simulink model "DS_distrIntp_4_0_realaxes"  (R2019b)
settings: Solver=FixedStepDiscrete  StartTime=0.0  StopTime=inf  FixedStep=Ts  RelTol=1e-3
StartFcn:
  | close all;
model workspace (MAT data in the model file):
  MvmtPerfEval_collectVal = Simulink.Parameter
  MvmtPerfEval_collectVal.Value = 0.65
  MvmtPerfEval_collectVal.Description = '- Anteil eines Interpolationssegments (0,1)
    | - Nach Abarbeitung des spezifizierten Anteils wird gemeinsame Performance aller Agenten
    | vom Dispatcher geladen
    | 
    | - (!!!) Wert MUSS größer sein als MvmtPerfEval_sendOwnVal'
  MvmtPerfEval_collectVal.DataType = 'auto'
  MvmtPerfEval_collectVal.Min = 0
  MvmtPerfEval_collectVal.Max = 1
  MvmtPerfEval_collectVal.Dimensions = [1 1]
  MvmtPerfEval_sendOwnVal = Simulink.Parameter
  MvmtPerfEval_sendOwnVal.Value = 0.6
  MvmtPerfEval_sendOwnVal.Description = '- Anteil eines Interpolationssegments (0,1)
    | - Nach Abarbeitung des spezifizierten Anteils wird Perfomance Kennzahl an Dispatcher übermittelt
    | 
    | - (!!!) Wert MUSS kleiner sein als MvmtPerfEval_collectVal'
  MvmtPerfEval_sendOwnVal.DataType = 'auto'
  MvmtPerfEval_sendOwnVal.Min = 0
  MvmtPerfEval_sendOwnVal.Max = 1
  MvmtPerfEval_sendOwnVal.Dimensions = [1 1]
  PAR_center_c2 = Simulink.Parameter
  PAR_center_c2.Value = [0.0775 0.062 0.05]
  PAR_center_c2.DataType = 'double'
  PAR_center_c2.Dimensions = [1 3]
  PAR_numStepsAheadSmoothing = Simulink.Parameter
  PAR_numStepsAheadSmoothing.Value = 1
  PAR_numStepsAheadSmoothing.Description = 'Anzahl der Zeitschritte (Ts) vor Segmentende, welches Zeitpunkt festlegt,
    | an dem der kommende Verfahrbefehl gesendet wird'
  PAR_numStepsAheadSmoothing.DataType = 'auto'
  PAR_numStepsAheadSmoothing.Dimensions = [1 1]
  PAR_startPosReachedTol = Simulink.Parameter
  PAR_startPosReachedTol.Value = 0.002
  PAR_startPosReachedTol.DataType = 'auto'
  PAR_startPosReachedTol.Dimensions = [1 1]
  PAR_workspace_c2 = Simulink.Parameter
  PAR_workspace_c2.Value = [0 0 0.05 0.052 0.072]
  PAR_workspace_c2.DataType = 'double'
  PAR_workspace_c2.Dimensions = [1 5]
  PerfEval_numTicks_enable = Simulink.Parameter
  PerfEval_numTicks_enable.Value = 10
  PerfEval_numTicks_enable.Description = 'Anzahl der Ticks (Integrationsschritte), bevor die Performance ausgewertet wird
    | (unabhängig vom Senden des Werts an den Dispatcher)'
  PerfEval_numTicks_enable.DataType = 'auto'
  PerfEval_numTicks_enable.Dimensions = [1 1]
  Segmentregler_I_Gain = Simulink.Parameter
  Segmentregler_I_Gain.Value = 1
  Segmentregler_I_Gain.DataType = 'auto'
  Segmentregler_I_Gain.Dimensions = [1 1]
  Segmentregler_P_Gain = Simulink.Parameter
  Segmentregler_P_Gain.Value = 0
  Segmentregler_P_Gain.DataType = 'auto'
  Segmentregler_P_Gain.Dimensions = [1 1]
  Segmentregler_minVel_enable = Simulink.Parameter
  Segmentregler_minVel_enable.Value = 0.1
  Segmentregler_minVel_enable.DataType = 'auto'
  Segmentregler_minVel_enable.Dimensions = [1 1]
  Segmentregler_numTicks_enable = Simulink.Parameter
  Segmentregler_numTicks_enable.Value = 30
  Segmentregler_numTicks_enable.Description = 'Anzahl der Ticks (Integrationsschritte), bevor der Segmentregler aktiv wird'
  Segmentregler_numTicks_enable.DataType = 'auto'
  Segmentregler_numTicks_enable.Dimensions = [1 1]
  Ts = Simulink.Parameter
  Ts.Value = 0.005
  Ts.Description = 'Sampling Time'
  Ts.DataType = 'auto'
  Ts.Dimensions = [1 1]
  horizon = Simulink.Parameter
  horizon.Value = 0
  horizon.DataType = 'auto'
  horizon.Dimensions = [1 1]
  maxPos_x = Simulink.Parameter
  maxPos_x.Value = 300
  maxPos_x.Description = 'Grenze des Arbeitsbereichs (maximaler Wert der Koordinate)'
  maxPos_x.DataType = 'auto'
  maxPos_x.Dimensions = [1 1]
  maxPos_y = Simulink.Parameter
  maxPos_y.Value = 150
  maxPos_y.Description = 'Grenze des Arbeitsbereichs (maximaler Wert der Koordinate)'
  maxPos_y.DataType = 'auto'
  maxPos_y.Dimensions = [1 1]
  maxPos_z = Simulink.Parameter
  maxPos_z.Value = 50
  maxPos_z.Description = 'Grenze des Arbeitsbereichs (maximaler Wert der Koordinate)'
  maxPos_z.DataType = 'auto'
  maxPos_z.Dimensions = [1 1]
  maxVectorLengths = Simulink.Parameter
  maxVectorLengths.Value = 100000
  maxVectorLengths.DataType = 'auto'
  maxVectorLengths.Dimensions = [1 1]
  minAllowedVelSaturation = Simulink.Parameter
  minAllowedVelSaturation.Value = 0.25
  minAllowedVelSaturation.Description = 'Minimaler Saturation-Wert für den Geschwindigkeits-PID-Regler
    | (auch bei Sollgeschwindigkeit soll Fehlerkorrektur möglich sein)'
  minAllowedVelSaturation.DataType = 'auto'
  minAllowedVelSaturation.Dimensions = [1 1]
  numAxes = Simulink.Parameter
  numAxes.Value = 4
  numAxes.DataType = 'auto'
  numAxes.Dimensions = [1 1]
  window_length = Simulink.Parameter
  window_length.Value = 50
  window_length.DataType = 'auto'
  window_length.Dimensions = [1 1]
undefined symbols (not defined in the file or in its folder): DiscIntNeverNeededParam, setP_mat, VelOverride
libraries: vrlib x1, sldrtlib x1
(part 1 of 4)
settings Model: OrderedModelArguments=off  Creator=Daniel  LastModifiedBy=MAHFOUZ
settings DataIOCC: SignalLogging=off  ReturnWorkspaceOutputs=off
settings DebuggingCC: ArithmeticOperatorsInVariantConditions=warning
settings SFSimCC: CustomCodeUndefinedFunction=UseInterfaceOnly

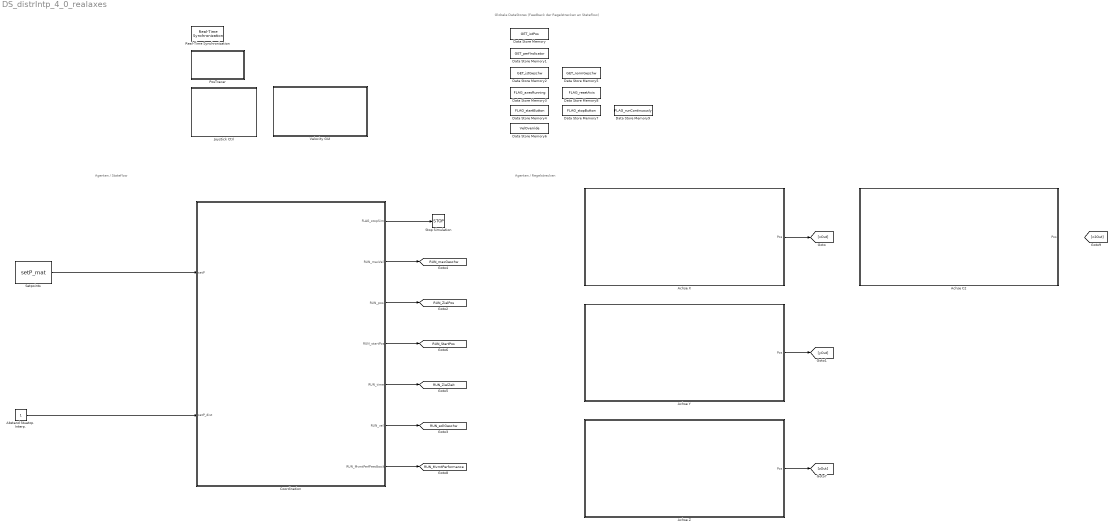
== system DS_distrIntp_4_0_realaxes ==
  note: Globale DataStores (Feedback der Regelstrecken an Stateflow)
  note: Agenten / Regelstrecken
  note: Agenten / Stateflow
  Abstand Stuetzp. Interp. : Constant
  Achse C2 : Subsystem
  Achse X : Subsystem
  Achse Y : Subsystem
  Achse Z : Subsystem
  Coordination : Stateflow chart  TreatAsAtomicUnit=on
  Data Store Memory : DataStoreMemory  DataStoreName=GET_istPos  ReadBeforeWriteMsg=warning  WriteAfterWriteMsg=warning  WriteAfterReadMsg=warning  InitialValue=zeros(1,numAxes)  ShowAdditionalParam=off  OutDataTypeStr=double
  Data Store Memory1 : DataStoreMemory  DataStoreName=GET_perfIndicator  ReadBeforeWriteMsg=warning  WriteAfterWriteMsg=warning  WriteAfterReadMsg=warning  InitialValue=zeros(1,numAxes)  ShowAdditionalParam=off  OutDataTypeStr=double
  Data Store Memory2 : DataStoreMemory  DataStoreName=GET_istGeschw  ReadBeforeWriteMsg=warning  WriteAfterWriteMsg=warning  WriteAfterReadMsg=warning  InitialValue=zeros(1,numAxes)  ShowAdditionalParam=off  OutDataTypeStr=double
  Data Store Memory3 : DataStoreMemory  DataStoreName=FLAG_axesRunning  ReadBeforeWriteMsg=warning  WriteAfterWriteMsg=warning  WriteAfterReadMsg=warning  InitialValue=false  ShowAdditionalParam=off  OutDataTypeStr=boolean
  Data Store Memory4 : DataStoreMemory  DataStoreName=FLAG_startButton  ReadBeforeWriteMsg=warning  WriteAfterWriteMsg=warning  WriteAfterReadMsg=warning  InitialValue=false  ShowAdditionalParam=off  OutDataTypeStr=boolean
  Data Store Memory5 : DataStoreMemory  DataStoreName=GET_normGeschw  ReadBeforeWriteMsg=warning  WriteAfterWriteMsg=warning  WriteAfterReadMsg=warning  InitialValue=zeros(1,numAxes)  ShowAdditionalParam=off  OutDataTypeStr=double
  Data Store Memory6 : DataStoreMemory  DataStoreName=VelOverride  ReadBeforeWriteMsg=warning  WriteAfterWriteMsg=warning  WriteAfterReadMsg=warning  InitialValue=ones(1,numAxes)  ShowAdditionalParam=off  OutDataTypeStr=double
  Data Store Memory7 : DataStoreMemory  DataStoreName=FLAG_stopButton  ReadBeforeWriteMsg=warning  WriteAfterWriteMsg=warning  WriteAfterReadMsg=warning  InitialValue=false  ShowAdditionalParam=off  OutDataTypeStr=boolean
  Data Store Memory8 : DataStoreMemory  DataStoreName=FLAG_resetAxis  ReadBeforeWriteMsg=warning  WriteAfterWriteMsg=warning  WriteAfterReadMsg=warning  InitialValue=zeros(1,numAxes)  ShowAdditionalParam=off  OutDataTypeStr=boolean
  Data Store Memory9 : DataStoreMemory  DataStoreName=FLAG_runContinuously  ReadBeforeWriteMsg=warning  WriteAfterWriteMsg=warning  WriteAfterReadMsg=warning  ShowAdditionalParam=off  OutDataTypeStr=double
  Joystick Ctrl : Subsystem
  PosTracer : Stateflow chart  BlockKeywords=__PRM__SERIALIZED__DATA__:Stateflow Chart,Stateflow Diagram  TreatAsAtomicUnit=on
  Real-Time Synchronization : sldrtlib/Real-Time Synchronization  SampleTime=0.005  MaxMissedTicks=2000  ShowMissedTicks=off  YieldWhenWaiting=off
  Setpoints : Constant  Value=setP_mat
  Stop Simulation : Stop
  Velocity GUI : Subsystem
  tag scope: RUN_MvmtPerformance=global, RUN_StartPos=global, RUN_ZielPos=global, RUN_ZielZeit=global, RUN_maxGeschw=global, RUN_sollGeschw=global
  wires:
  Abstand Stuetzp. Interp./1 -> Coordination/2(setP_dist)
  Setpoints/1 -> Coordination/1(setP)
  Coordination/2(RUN_maxVel) -> [RUN_maxGeschw]
  Coordination/3(RUN_pos) -> [RUN_ZielPos]
  Coordination/4(RUN_startPos) -> [RUN_StartPos]
  Coordination/5(RUN_time) -> [RUN_ZielZeit]
  Coordination/6(RUN_vel) -> [RUN_sollGeschw]
  Achse Z/1(Pos) -> [zOut]
  Coordination/7(RUN_MvmtPerfFeedback) -> [RUN_MvmtPerformance]
  Achse X/1(Pos) -> [xOut]
  Achse Y/1(Pos) -> [yOut]
  ? -> [c2Out]
  Coordination/1(FLAG_stopSim) -> Stop Simulation/1

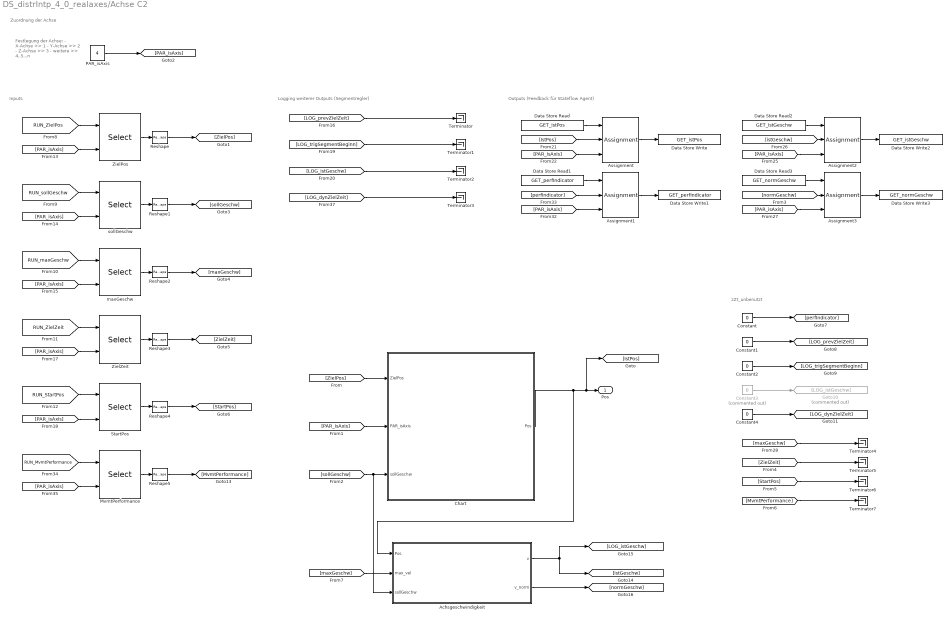
== system DS_distrIntp_4_0_realaxes/Achse C2 ==
  note: Outputs (Feedback für Stateflow Agent)
  note: Logging weiterer Outputs (Segmentregler)
  note: Zuordnung der Achse
  note: Festlegung der Achse:
      | - X-Achse >> 1
      | - Y-Achse >> 2
      | - Z-Achse >> 3
      | - weitere >> 4..5...n
  note: Inputs
  note: zZt_unbenutzt
  Achsgeschwindigkeit : Stateflow chart  BlockKeywords=__PRM__SERIALIZED__DATA__:Stateflow Chart,Stateflow Diagram  TreatAsAtomicUnit=on
  Assignment{,1..3} (4 alike) : Assignment  DiagnosticForDimensions=Warning  IndexOptions=Index vector (port)  Indices=1  OutputSizes=1
  Chart : Stateflow chart  BlockKeywords=__PRM__SERIALIZED__DATA__:Stateflow Chart,Stateflow Diagram  TreatAsAtomicUnit=on
  Constant{,1..2,4} (4 alike) : Constant  Value=0
  Constant3 : Constant  Commented=on  Value=0
  Data Store Read : DataStoreRead  DataStoreName=GET_istPos
  Data Store Read1 : DataStoreRead  DataStoreName=GET_perfIndicator
  Data Store Read2 : DataStoreRead  DataStoreName=GET_istGeschw
  Data Store Read3 : DataStoreRead  DataStoreName=GET_normGeschw
  Data Store Write : DataStoreWrite  DataStoreName=GET_istPos
  Data Store Write1 : DataStoreWrite  DataStoreName=GET_perfIndicator
  Data Store Write2 : DataStoreWrite  DataStoreName=GET_istGeschw
  Data Store Write3 : DataStoreWrite  DataStoreName=GET_normGeschw
  Goto10 : Goto  Commented=on  GotoTag=LOG_istGeschw
  MvmtPerformance : Selector  IndexOptions=Index vector (port)  Indices=[1 3]  OutputSizes=1
  PAR_isAxis : Constant  Value=4
  Reshape{,1..5} (6 alike) : Reshape
  StartPos : Selector  IndexOptions=Index vector (port)  Indices=[1 3]  OutputSizes=1
  Terminator{,1..7} (8 alike) : Terminator
  ZielPos : Selector  IndexOptions=Index vector (port)  Indices=[1 3]  OutputSizes=1
  ZielZeit : Selector  IndexOptions=Index vector (port)  Indices=[1 3]  OutputSizes=1
  maxGeschw : Selector  IndexOptions=Index vector (port)  Indices=[1 3]  OutputSizes=1
  sollGeschw : Selector  IndexOptions=Index vector (port)  Indices=[1 3]  OutputSizes=1
  Pos : Outport  VectorParamsAs1DForOutWhenUnconnected=off
  wires:
  PAR_isAxis/1 -> [PAR_isAxis]
  [PAR_isAxis] -> ZielPos/2
  [RUN_ZielPos] -> ZielPos/1
  ZielPos/1 -> Reshape/1
  sollGeschw/1 -> Reshape1/1
  [RUN_sollGeschw] -> sollGeschw/1
  [PAR_isAxis] -> sollGeschw/2
  [PAR_isAxis] -> maxGeschw/2
  [RUN_maxGeschw] -> maxGeschw/1
  maxGeschw/1 -> Reshape2/1
  ZielZeit/1 -> Reshape3/1
  [RUN_ZielZeit] -> ZielZeit/1
  [PAR_isAxis] -> ZielZeit/2
  [PAR_isAxis] -> StartPos/2
  [RUN_StartPos] -> StartPos/1
  StartPos/1 -> Reshape4/1
  [LOG_prevZielZeit] -> Terminator/1
  [LOG_trigSegmentBeginn] -> Terminator1/1
  [LOG_istGeschw] -> Terminator2/1
  Reshape/1 -> [ZielPos]
  Reshape1/1 -> [sollGeschw]
  Reshape2/1 -> [maxGeschw]
  Reshape4/1 -> [StartPos]
  Reshape3/1 -> [ZielZeit]
  Data Store Read/1 -> Assignment/1
  [IstPos] -> Assignment/2
  [PAR_isAxis] -> Assignment/3
  Assignment/1 -> Data Store Write/1
  Assignment1/1 -> Data Store Write1/1
  [PAR_isAxis] -> Assignment1/3
  [perfIndicator] -> Assignment1/2
  Data Store Read1/1 -> Assignment1/1
  Reshape5/1 -> [MvmtPerformance]
  MvmtPerformance/1 -> Reshape5/1
  [RUN_MvmtPerformance] -> MvmtPerformance/1
  [PAR_isAxis] -> MvmtPerformance/2
  [LOG_dynZielZeit] -> Terminator3/1
  Constant4/1 -> [LOG_dynZielZeit]
  Constant1/1 -> [LOG_prevZielZeit]
  [StartPos] -> Terminator6/1
  Constant2/1 -> [LOG_trigSegmentBeginn]
  [ZielZeit] -> Terminator5/1
  Constant/1 -> [perfIndicator]
  Constant3/1 -> Goto10/1
  [maxGeschw] -> Terminator4/1
  [MvmtPerformance] -> Terminator7/1
  [ZielPos] -> Chart/1(ZielPos)
  [PAR_isAxis] -> Chart/2(PAR_isAxis)
  [sollGeschw] -> Achsgeschwindigkeit/3(sollGeschw), Chart/3(sollGeschw)
  Chart/1(Pos) -> Achsgeschwindigkeit/1(Pos), Pos/1, [IstPos]
  Achsgeschwindigkeit/1(v) -> [istGeschw], [LOG_istGeschw]
  [normGeschw] -> Assignment3/2
  [istGeschw] -> Assignment2/2
  [PAR_isAxis] -> Assignment2/3
  [PAR_isAxis] -> Assignment3/3
  Assignment3/1 -> Data Store Write3/1
  Assignment2/1 -> Data Store Write2/1
  Data Store Read2/1 -> Assignment2/1
  Data Store Read3/1 -> Assignment3/1
  Achsgeschwindigkeit/2(v_norm) -> [normGeschw]
  [maxGeschw] -> Achsgeschwindigkeit/2(max_vel)

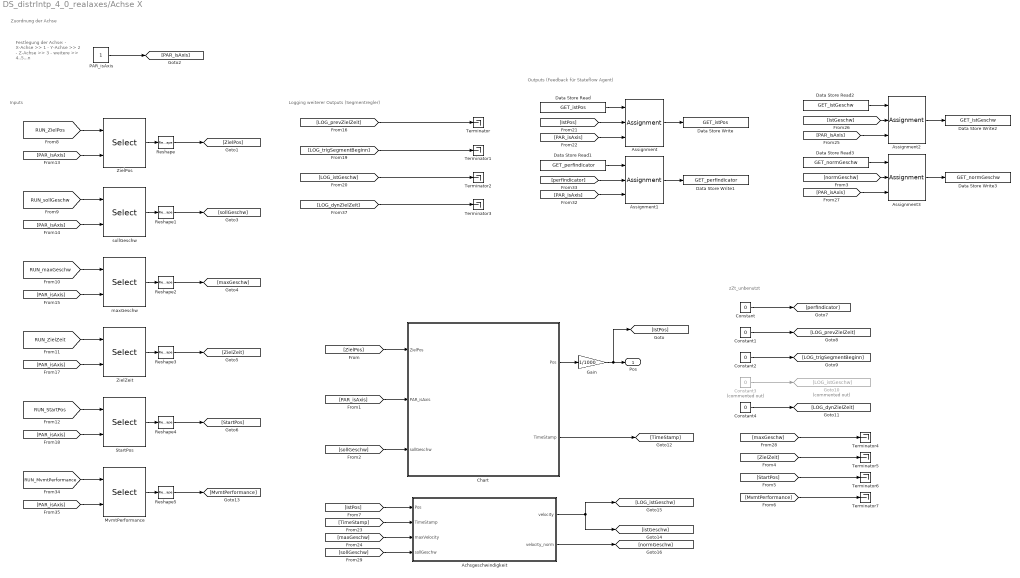
== system DS_distrIntp_4_0_realaxes/Achse X ==
  note: zZt_unbenutzt
  note: Outputs (Feedback für Stateflow Agent)
  note: Logging weiterer Outputs (Segmentregler)
  note: Zuordnung der Achse
  note: Festlegung der Achse:
      | - X-Achse >> 1
      | - Y-Achse >> 2
      | - Z-Achse >> 3
      | - weitere >> 4..5...n
  note: Inputs
  Achsgeschwindigkeit : Stateflow chart  BlockKeywords=__PRM__SERIALIZED__DATA__:Stateflow Chart,Stateflow Diagram  TreatAsAtomicUnit=on
  Assignment{,1..3} (4 alike) : Assignment  DiagnosticForDimensions=Warning  IndexOptions=Index vector (port)  Indices=1  OutputSizes=1
  Chart : Stateflow chart  BlockKeywords=__PRM__SERIALIZED__DATA__:Stateflow Chart,Stateflow Diagram  TreatAsAtomicUnit=on
  Constant{,1..2,4} (4 alike) : Constant  Value=0
  Constant3 : Constant  Commented=on  Value=0
  Data Store Read : DataStoreRead  DataStoreName=GET_istPos
  Data Store Read1 : DataStoreRead  DataStoreName=GET_perfIndicator
  Data Store Read2 : DataStoreRead  DataStoreName=GET_istGeschw
  Data Store Read3 : DataStoreRead  DataStoreName=GET_normGeschw
  Data Store Write : DataStoreWrite  DataStoreName=GET_istPos
  Data Store Write1 : DataStoreWrite  DataStoreName=GET_perfIndicator
  Data Store Write2 : DataStoreWrite  DataStoreName=GET_istGeschw
  Data Store Write3 : DataStoreWrite  DataStoreName=GET_normGeschw
  Gain : Gain  Gain=1/1000
  Goto10 : Goto  Commented=on  GotoTag=LOG_istGeschw
  MvmtPerformance : Selector  IndexOptions=Index vector (port)  Indices=[1 3]  OutputSizes=1
  PAR_isAxis : Constant
  Reshape{,1..5} (6 alike) : Reshape
  StartPos : Selector  IndexOptions=Index vector (port)  Indices=[1 3]  OutputSizes=1
  Terminator{,1..7} (8 alike) : Terminator
  ZielPos : Selector  IndexOptions=Index vector (port)  Indices=[1 3]  OutputSizes=1
  ZielZeit : Selector  IndexOptions=Index vector (port)  Indices=[1 3]  OutputSizes=1
  maxGeschw : Selector  IndexOptions=Index vector (port)  Indices=[1 3]  OutputSizes=1
  sollGeschw : Selector  IndexOptions=Index vector (port)  Indices=[1 3]  OutputSizes=1
  Pos : Outport  VectorParamsAs1DForOutWhenUnconnected=off
  wires:
  Gain/1 -> Pos/1, [IstPos]
  PAR_isAxis/1 -> [PAR_isAxis]
  [PAR_isAxis] -> ZielPos/2
  [RUN_ZielPos] -> ZielPos/1
  ZielPos/1 -> Reshape/1
  sollGeschw/1 -> Reshape1/1
  [RUN_sollGeschw] -> sollGeschw/1
  [PAR_isAxis] -> sollGeschw/2
  [PAR_isAxis] -> maxGeschw/2
  [RUN_maxGeschw] -> maxGeschw/1
  maxGeschw/1 -> Reshape2/1
  ZielZeit/1 -> Reshape3/1
  [RUN_ZielZeit] -> ZielZeit/1
  [PAR_isAxis] -> ZielZeit/2
  [PAR_isAxis] -> StartPos/2
  [RUN_StartPos] -> StartPos/1
  StartPos/1 -> Reshape4/1
  [LOG_prevZielZeit] -> Terminator/1
  [LOG_trigSegmentBeginn] -> Terminator1/1
  [LOG_istGeschw] -> Terminator2/1
  Reshape/1 -> [ZielPos]
  Reshape1/1 -> [sollGeschw]
  Reshape2/1 -> [maxGeschw]
  Reshape4/1 -> [StartPos]
  Reshape3/1 -> [ZielZeit]
  Data Store Read/1 -> Assignment/1
  [IstPos] -> Assignment/2
  [PAR_isAxis] -> Assignment/3
  Assignment/1 -> Data Store Write/1
  Assignment1/1 -> Data Store Write1/1
  [PAR_isAxis] -> Assignment1/3
  [perfIndicator] -> Assignment1/2
  Data Store Read1/1 -> Assignment1/1
  Reshape5/1 -> [MvmtPerformance]
  MvmtPerformance/1 -> Reshape5/1
  [RUN_MvmtPerformance] -> MvmtPerformance/1
  [PAR_isAxis] -> MvmtPerformance/2
  [LOG_dynZielZeit] -> Terminator3/1
  [ZielPos] -> Chart/1(ZielPos)
  [PAR_isAxis] -> Chart/2(PAR_isAxis)
  [sollGeschw] -> Chart/3(sollGeschw)
  Constant/1 -> [perfIndicator]
  Constant1/1 -> [LOG_prevZielZeit]
  Constant2/1 -> [LOG_trigSegmentBeginn]
  Constant3/1 -> Goto10/1
  Constant4/1 -> [LOG_dynZielZeit]
  [ZielZeit] -> Terminator5/1
  [StartPos] -> Terminator6/1
  [MvmtPerformance] -> Terminator7/1
  Chart/1(Pos) -> Gain/1
  [IstPos] -> Achsgeschwindigkeit/1(Pos)
  Chart/2(TimeStamp) -> [TimeStamp]
  [TimeStamp] -> Achsgeschwindigkeit/2(TimeStamp)
  Achsgeschwindigkeit/1(velocity) -> [LOG_istGeschw], [istGeschw]
  Assignment2/1 -> Data Store Write2/1
  [PAR_isAxis] -> Assignment2/3
  Data Store Read2/1 -> Assignment2/1
  [istGeschw] -> Assignment2/2
  [maxGeschw] -> Achsgeschwindigkeit/3(maxVelocity)
  [PAR_isAxis] -> Assignment3/3
  Assignment3/1 -> Data Store Write3/1
  Data Store Read3/1 -> Assignment3/1
  Achsgeschwindigkeit/2(velocity_norm) -> [normGeschw]
  [normGeschw] -> Assignment3/2
  [maxGeschw] -> Terminator4/1
  [sollGeschw] -> Achsgeschwindigkeit/4(sollGeschw)

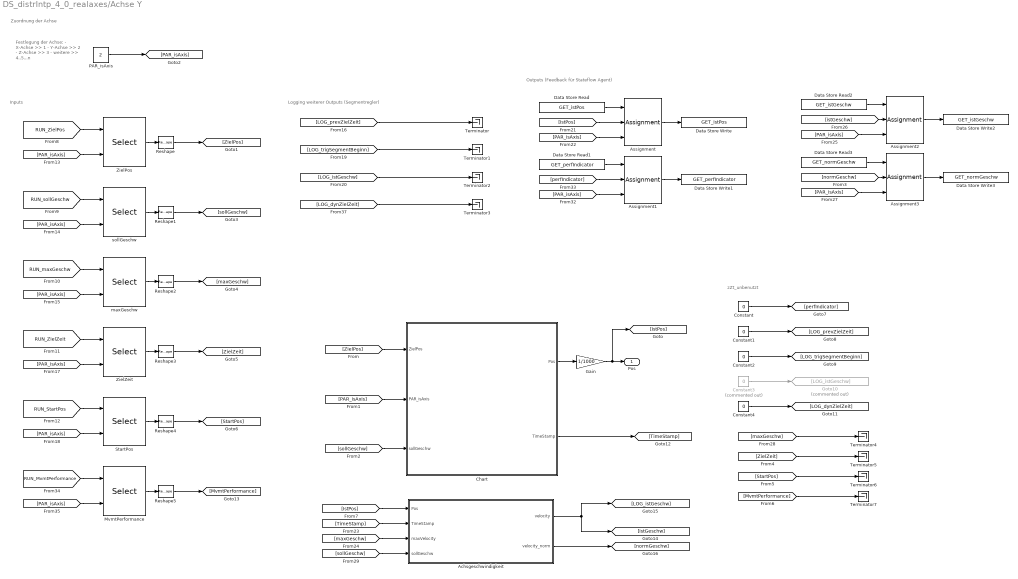
== system DS_distrIntp_4_0_realaxes/Achse Y ==
  note: Inputs
  note: Festlegung der Achse:
      | - X-Achse >> 1
      | - Y-Achse >> 2
      | - Z-Achse >> 3
      | - weitere >> 4..5...n
  note: Zuordnung der Achse
  note: Logging weiterer Outputs (Segmentregler)
  note: Outputs (Feedback für Stateflow Agent)
  note: zZt_unbenutzt
  Achsgeschwindigkeit : Stateflow chart  BlockKeywords=__PRM__SERIALIZED__DATA__:Stateflow Chart,Stateflow Diagram  TreatAsAtomicUnit=on
  Assignment{,1..3} (4 alike) : Assignment  DiagnosticForDimensions=Warning  IndexOptions=Index vector (port)  Indices=1  OutputSizes=1
  Chart : Stateflow chart  BlockKeywords=__PRM__SERIALIZED__DATA__:Stateflow Chart,Stateflow Diagram  TreatAsAtomicUnit=on
  Constant{,1..2,4} (4 alike) : Constant  Value=0
  Constant3 : Constant  Commented=on  Value=0
  Data Store Read : DataStoreRead  DataStoreName=GET_istPos
  Data Store Read1 : DataStoreRead  DataStoreName=GET_perfIndicator
  Data Store Read2 : DataStoreRead  DataStoreName=GET_istGeschw
  Data Store Read3 : DataStoreRead  DataStoreName=GET_normGeschw
  Data Store Write : DataStoreWrite  DataStoreName=GET_istPos
  Data Store Write1 : DataStoreWrite  DataStoreName=GET_perfIndicator
  Data Store Write2 : DataStoreWrite  DataStoreName=GET_istGeschw
  Data Store Write3 : DataStoreWrite  DataStoreName=GET_normGeschw
  Gain : Gain  Gain=1/1000
  Goto10 : Goto  Commented=on  GotoTag=LOG_istGeschw
  MvmtPerformance : Selector  IndexOptions=Index vector (port)  Indices=[1 3]  OutputSizes=1
  PAR_isAxis : Constant  Value=2
  Reshape{,1..5} (6 alike) : Reshape
  StartPos : Selector  IndexOptions=Index vector (port)  Indices=[1 3]  OutputSizes=1
  Terminator{,1..7} (8 alike) : Terminator
  ZielPos : Selector  IndexOptions=Index vector (port)  Indices=[1 3]  OutputSizes=1
  ZielZeit : Selector  IndexOptions=Index vector (port)  Indices=[1 3]  OutputSizes=1
  maxGeschw : Selector  IndexOptions=Index vector (port)  Indices=[1 3]  OutputSizes=1
  sollGeschw : Selector  IndexOptions=Index vector (port)  Indices=[1 3]  OutputSizes=1
  Pos : Outport  VectorParamsAs1DForOutWhenUnconnected=off
  wires:
  [maxGeschw] -> Terminator4/1
  [normGeschw] -> Assignment3/2
  Data Store Read3/1 -> Assignment3/1
  Assignment3/1 -> Data Store Write3/1
  [PAR_isAxis] -> Assignment3/3
  [istGeschw] -> Assignment2/2
  Data Store Read2/1 -> Assignment2/1
  [PAR_isAxis] -> Assignment2/3
  Assignment2/1 -> Data Store Write2/1
  Chart/2(TimeStamp) -> [TimeStamp]
  Chart/1(Pos) -> Gain/1
  [MvmtPerformance] -> Terminator7/1
  [StartPos] -> Terminator6/1
  [ZielZeit] -> Terminator5/1
  Constant4/1 -> [LOG_dynZielZeit]
  Constant3/1 -> Goto10/1
  Constant2/1 -> [LOG_trigSegmentBeginn]
  Constant1/1 -> [LOG_prevZielZeit]
  Constant/1 -> [perfIndicator]
  [sollGeschw] -> Chart/3(sollGeschw)
  [PAR_isAxis] -> Chart/2(PAR_isAxis)
  [ZielPos] -> Chart/1(ZielPos)
  [LOG_dynZielZeit] -> Terminator3/1
  [PAR_isAxis] -> MvmtPerformance/2
  [RUN_MvmtPerformance] -> MvmtPerformance/1
  MvmtPerformance/1 -> Reshape5/1
  Reshape5/1 -> [MvmtPerformance]
  Data Store Read1/1 -> Assignment1/1
  [perfIndicator] -> Assignment1/2
  [PAR_isAxis] -> Assignment1/3
  Assignment1/1 -> Data Store Write1/1
  Assignment/1 -> Data Store Write/1
  [PAR_isAxis] -> Assignment/3
  [IstPos] -> Assignment/2
  Data Store Read/1 -> Assignment/1
  Reshape3/1 -> [ZielZeit]
  Reshape4/1 -> [StartPos]
  Reshape2/1 -> [maxGeschw]
  Reshape1/1 -> [sollGeschw]
  Reshape/1 -> [ZielPos]
  [LOG_istGeschw] -> Terminator2/1
  [LOG_trigSegmentBeginn] -> Terminator1/1
  [LOG_prevZielZeit] -> Terminator/1
  StartPos/1 -> Reshape4/1
  [RUN_StartPos] -> StartPos/1
  [PAR_isAxis] -> StartPos/2
  [PAR_isAxis] -> ZielZeit/2
  [RUN_ZielZeit] -> ZielZeit/1
  ZielZeit/1 -> Reshape3/1
  maxGeschw/1 -> Reshape2/1
  [RUN_maxGeschw] -> maxGeschw/1
  [PAR_isAxis] -> maxGeschw/2
  [PAR_isAxis] -> sollGeschw/2
  [RUN_sollGeschw] -> sollGeschw/1
  sollGeschw/1 -> Reshape1/1
  ZielPos/1 -> Reshape/1
  [RUN_ZielPos] -> ZielPos/1
  [PAR_isAxis] -> ZielPos/2
  PAR_isAxis/1 -> [PAR_isAxis]
  Gain/1 -> [IstPos], Pos/1
  [maxGeschw] -> Achsgeschwindigkeit/3(maxVelocity)
  Achsgeschwindigkeit/1(velocity) -> [LOG_istGeschw], [istGeschw]
  Achsgeschwindigkeit/2(velocity_norm) -> [normGeschw]
  [IstPos] -> Achsgeschwindigkeit/1(Pos)
  [TimeStamp] -> Achsgeschwindigkeit/2(TimeStamp)
  [sollGeschw] -> Achsgeschwindigkeit/4(sollGeschw)

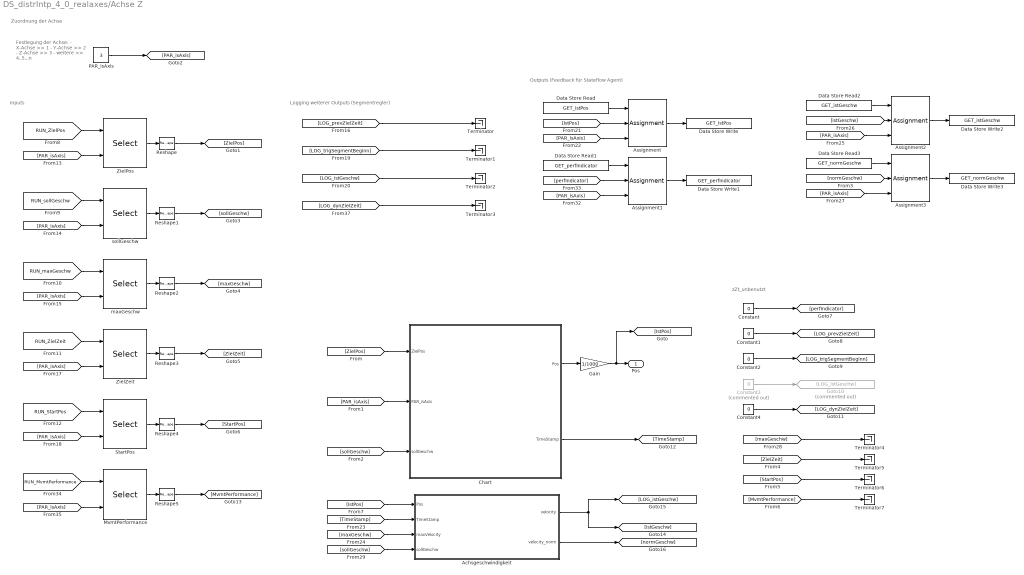
== system DS_distrIntp_4_0_realaxes/Achse Z ==
  note: zZt_unbenutzt
  note: Outputs (Feedback für Stateflow Agent)
  note: Logging weiterer Outputs (Segmentregler)
  note: Zuordnung der Achse
  note: Festlegung der Achse:
      | - X-Achse >> 1
      | - Y-Achse >> 2
      | - Z-Achse >> 3
      | - weitere >> 4..5...n
  note: Inputs
  Achsgeschwindigkeit : Stateflow chart  BlockKeywords=__PRM__SERIALIZED__DATA__:Stateflow Chart,Stateflow Diagram  TreatAsAtomicUnit=on
  Assignment{,1..3} (4 alike) : Assignment  DiagnosticForDimensions=Warning  IndexOptions=Index vector (port)  Indices=1  OutputSizes=1
  Chart : Stateflow chart  BlockKeywords=__PRM__SERIALIZED__DATA__:Stateflow Chart,Stateflow Diagram  TreatAsAtomicUnit=on
  Constant{,1..2,4} (4 alike) : Constant  Value=0
  Constant3 : Constant  Commented=on  Value=0
  Data Store Read : DataStoreRead  DataStoreName=GET_istPos
  Data Store Read1 : DataStoreRead  DataStoreName=GET_perfIndicator
  Data Store Read2 : DataStoreRead  DataStoreName=GET_istGeschw
  Data Store Read3 : DataStoreRead  DataStoreName=GET_normGeschw
  Data Store Write : DataStoreWrite  DataStoreName=GET_istPos
  Data Store Write1 : DataStoreWrite  DataStoreName=GET_perfIndicator
  Data Store Write2 : DataStoreWrite  DataStoreName=GET_istGeschw
  Data Store Write3 : DataStoreWrite  DataStoreName=GET_normGeschw
  Gain : Gain  Gain=1/1000
  Goto10 : Goto  Commented=on  GotoTag=LOG_istGeschw
  MvmtPerformance : Selector  IndexOptions=Index vector (port)  Indices=[1 3]  OutputSizes=1
  PAR_isAxis : Constant  Value=3
  Reshape{,1..5} (6 alike) : Reshape
  StartPos : Selector  IndexOptions=Index vector (port)  Indices=[1 3]  OutputSizes=1
  Terminator{,1..7} (8 alike) : Terminator
  ZielPos : Selector  IndexOptions=Index vector (port)  Indices=[1 3]  OutputSizes=1
  ZielZeit : Selector  IndexOptions=Index vector (port)  Indices=[1 3]  OutputSizes=1
  maxGeschw : Selector  IndexOptions=Index vector (port)  Indices=[1 3]  OutputSizes=1
  sollGeschw : Selector  IndexOptions=Index vector (port)  Indices=[1 3]  OutputSizes=1
  Pos : Outport  VectorParamsAs1DForOutWhenUnconnected=off
  wires:
  Gain/1 -> Pos/1, [IstPos]
  PAR_isAxis/1 -> [PAR_isAxis]
  [PAR_isAxis] -> ZielPos/2
  [RUN_ZielPos] -> ZielPos/1
  ZielPos/1 -> Reshape/1
  sollGeschw/1 -> Reshape1/1
  [RUN_sollGeschw] -> sollGeschw/1
  [PAR_isAxis] -> sollGeschw/2
  [PAR_isAxis] -> maxGeschw/2
  [RUN_maxGeschw] -> maxGeschw/1
  maxGeschw/1 -> Reshape2/1
  ZielZeit/1 -> Reshape3/1
  [RUN_ZielZeit] -> ZielZeit/1
  [PAR_isAxis] -> ZielZeit/2
  [PAR_isAxis] -> StartPos/2
  [RUN_StartPos] -> StartPos/1
  StartPos/1 -> Reshape4/1
  [LOG_prevZielZeit] -> Terminator/1
  [LOG_trigSegmentBeginn] -> Terminator1/1
  [LOG_istGeschw] -> Terminator2/1
  Reshape/1 -> [ZielPos]
  Reshape1/1 -> [sollGeschw]
  Reshape2/1 -> [maxGeschw]
  Reshape4/1 -> [StartPos]
  Reshape3/1 -> [ZielZeit]
  Data Store Read/1 -> Assignment/1
  [IstPos] -> Assignment/2
  [PAR_isAxis] -> Assignment/3
  Assignment/1 -> Data Store Write/1
  Assignment1/1 -> Data Store Write1/1
  [PAR_isAxis] -> Assignment1/3
  [perfIndicator] -> Assignment1/2
  Data Store Read1/1 -> Assignment1/1
  Reshape5/1 -> [MvmtPerformance]
  MvmtPerformance/1 -> Reshape5/1
  [RUN_MvmtPerformance] -> MvmtPerformance/1
  [PAR_isAxis] -> MvmtPerformance/2
  [LOG_dynZielZeit] -> Terminator3/1
  [ZielPos] -> Chart/1(ZielPos)
  [PAR_isAxis] -> Chart/2(PAR_isAxis)
  [sollGeschw] -> Chart/3(sollGeschw)
  Constant/1 -> [perfIndicator]
  Constant1/1 -> [LOG_prevZielZeit]
  Constant2/1 -> [LOG_trigSegmentBeginn]
  Constant3/1 -> Goto10/1
  Constant4/1 -> [LOG_dynZielZeit]
  [ZielZeit] -> Terminator5/1
  [StartPos] -> Terminator6/1
  [MvmtPerformance] -> Terminator7/1
  Chart/1(Pos) -> Gain/1
  Chart/2(TimeStamp) -> [TimeStamp]
  Assignment2/1 -> Data Store Write2/1
  [PAR_isAxis] -> Assignment2/3
  Data Store Read2/1 -> Assignment2/1
  [istGeschw] -> Assignment2/2
  [PAR_isAxis] -> Assignment3/3
  Assignment3/1 -> Data Store Write3/1
  Data Store Read3/1 -> Assignment3/1
  [normGeschw] -> Assignment3/2
  [maxGeschw] -> Terminator4/1
  [maxGeschw] -> Achsgeschwindigkeit/3(maxVelocity)
  Achsgeschwindigkeit/1(velocity) -> [LOG_istGeschw], [istGeschw]
  Achsgeschwindigkeit/2(velocity_norm) -> [normGeschw]
  [IstPos] -> Achsgeschwindigkeit/1(Pos)
  [TimeStamp] -> Achsgeschwindigkeit/2(TimeStamp)
  [sollGeschw] -> Achsgeschwindigkeit/4(sollGeschw)

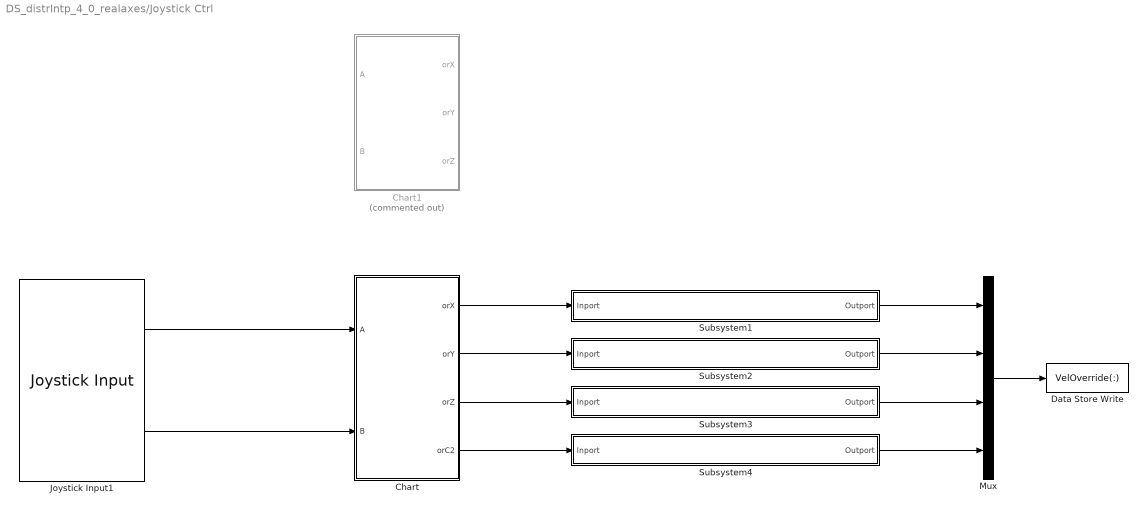
== system DS_distrIntp_4_0_realaxes/Joystick Ctrl ==
  Chart : Stateflow chart  BlockKeywords=__PRM__SERIALIZED__DATA__:Stateflow Chart,Stateflow Diagram  TreatAsAtomicUnit=on
  Chart1 : Stateflow chart  Commented=on  BlockKeywords=__PRM__SERIALIZED__DATA__:Stateflow Chart,Stateflow Diagram  TreatAsAtomicUnit=on  SystemSampleTime=0.1
  Data Store Write : DataStoreWrite  DataStoreName=VelOverride  DataStoreElements=VelOverride(:)
  Joystick Input1 : vrlib/Joystick Input  joyid=1  adjustports=off  forcefeed=off
      settings: SourceProductName=Simulink
  Mux : Mux
  Subsystem1 : Subsystem
  Subsystem2 : Subsystem
  Subsystem3 : Subsystem
  Subsystem4 : Subsystem
  wires:
  Chart/2(orY) -> Subsystem2/1(Inport)
  Chart/3(orZ) -> Subsystem3/1(Inport)
  Chart/1(orX) -> Subsystem1/1(Inport)
  Joystick Input1/2 -> Chart/2(B)
  Joystick Input1/1 -> Chart/1(A)
  Subsystem1/1(Outport) -> Mux/1
  Subsystem2/1(Outport) -> Mux/2
  Subsystem3/1(Outport) -> Mux/3
  Mux/1 -> Data Store Write/1
  Chart/4(orC2) -> Subsystem4/1(Inport)
  Subsystem4/1(Outport) -> Mux/4
